simulink model "ask_demod_signum"  (R2018a)
settings: Solver=VariableStepAuto  StartTime=0.0  StopTime=10.0  RelTol=1e-3
libraries: commrandsrc3 x1
settings Model: Creator=hp  LastModifiedBy=hp

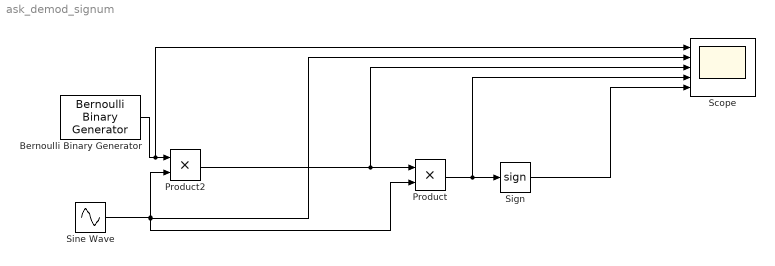
== system ask_demod_signum ==
  Bernoulli Binary Generator : commrandsrc3/Bernoulli Binary Generator  ProbabilityOfZero=0.3  SeedSource=Auto  Seed=0  SampleTime=1  SamplesPerFrame=1  OutputDataType=double  SimulateUsing=Interpreted execution
  Product : Product
  Product2 : Product
  Scope : Scope  NumInputPorts=5
  Sign : Signum
  Sine Wave : Sin  Frequency=2*pi*12  Samples=0.02  SampleTime=0.01
  wires:
  Bernoulli Binary Generator/1 -> Scope/1, Product2/1
  Sine Wave/1 -> Scope/2, Product/2, Product2/2
  Product2/1 -> Scope/3, Product/1
  Product/1 -> Scope/4, Sign/1
  Sign/1 -> Scope/5
